simulink model "untitled"  (R2025b)
settings: Solver=VariableStepAuto  StartTime=0.0  StopTime=10.0  RelTol=1e-3
settings Model: Creator=thomas-paulen  LastModifiedBy=thomas-paulen

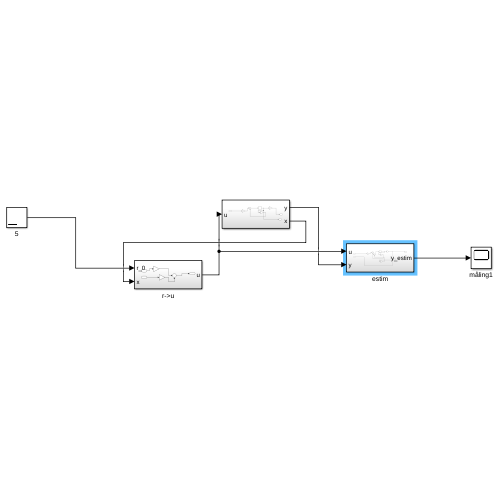
[thumbnail: Simulink's stored preview of the top-level diagram]
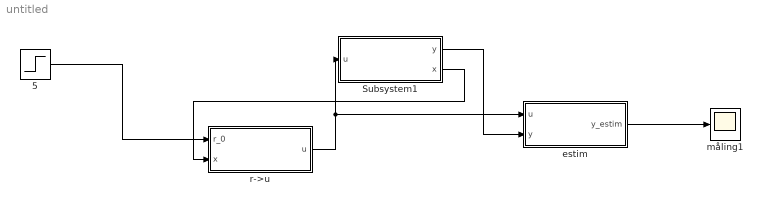
== system untitled ==
  5 : Step  After=5  SampleTime=0
  Subsystem1 : Subsystem
  estim : Subsystem
  måling1 : Scope
      settings: ActiveDisplayYMinimum=-0.62422868872445691  ActiveDisplayYMaximum=5.6180581985201137
  r->u : Subsystem
  wires:
  Subsystem1/1(y) -> estim/2(y)
  5/1 -> r->u/1(r_0)
  r->u/1(u) -> Subsystem1/1(u), estim/1(u)
  Subsystem1/2(x) -> r->u/2(x)
  estim/1(y_estim) -> måling1/1

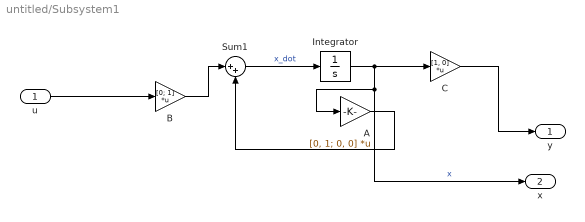
== system untitled/Subsystem1 ==
  u : Inport
  A : Gain  Gain=[0, 1; 0, 0]  Multiplication=Matrix(K*u)
  B : Gain  Gain=[0; 1]  Multiplication=Matrix(K*u)
  C : Gain  Gain=[1, 0]  Multiplication=Matrix(K*u)
  Integrator : Integrator
  Sum1 : Sum  Inputs=|++
  y : Outport
  x : Outport  Port=2
  wires:
  Integrator/1 -> C/1, x/1, A/1  "x"
  A/1 -> Sum1/2
  B/1 -> Sum1/1
  Sum1/1 -> Integrator/1  "x_dot"
  C/1 -> y/1
  u/1 -> B/1

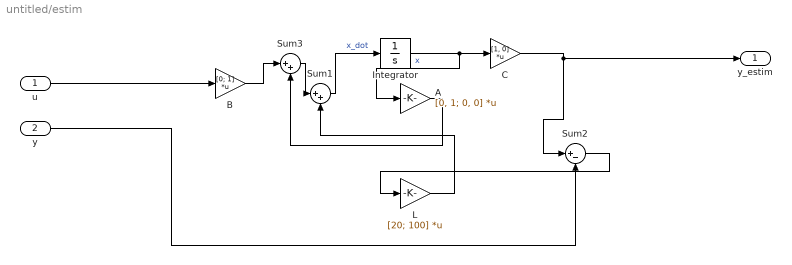
== system untitled/estim ==
  u : Inport
  y : Inport  Port=2
  A : Gain  Gain=[0, 1; 0, 0]  Multiplication=Matrix(K*u)
  B : Gain  Gain=[0; 1]  Multiplication=Matrix(K*u)
  C : Gain  Gain=[1, 0]  Multiplication=Matrix(K*u)
  Integrator : Integrator
  L : Gain  Gain=[20; 100]  Multiplication=Matrix(K*u)
  Sum1 : Sum  Inputs=|++
  Sum2 : Sum  Inputs=|+-
  Sum3 : Sum  Inputs=|++
  y_estim : Outport
  wires:
  Sum1/1 -> Integrator/1  "x_dot"
  Integrator/1 -> A/1, C/1  "x"
  B/1 -> Sum3/1
  C/1 -> Sum2/1, y_estim/1
  y/1 -> Sum2/2
  Sum2/1 -> L/1
  L/1 -> Sum1/2
  A/1 -> Sum3/2
  Sum3/1 -> Sum1/1
  u/1 -> B/1

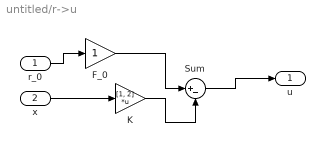
== system untitled/r->u ==
  r_0 : Inport
  x : Inport  Port=2
  F_0 : Gain
  K : Gain  Gain=[1, 2]  Multiplication=Matrix(K*u)
  Sum : Sum  Inputs=|+-
  u : Outport
  wires:
  x/1 -> K/1
  r_0/1 -> F_0/1
  F_0/1 -> Sum/1
  K/1 -> Sum/2
  Sum/1 -> u/1
